simulink model "test"  (R2013b)
settings: Solver=ode45  StartTime=0.0  StopTime=10  RelTol=1e-3
settings Model: Creator=Walter  LastModifiedBy=Walter
settings DataIOCC: SignalLoggingSaveFormat=ModelDataLogs
settings DebuggingCC: MultiTaskDSMMsg=warning  MultiTaskCondExecSysMsg=none
settings RTWCC: IncludeERTFirstTime=on

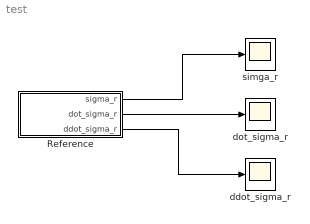
== system test ==
  Reference : Subsystem
  ddot_sigma_r : Scope
      settings: SaveName=ScopeData2
  dot_sigma_r : Scope
  simga_r : Scope
  wires:
  Reference/1(sigma_r) -> simga_r/1
  Reference/3(ddot_sigma_r) -> ddot_sigma_r/1
  Reference/2(dot_sigma_r) -> dot_sigma_r/1

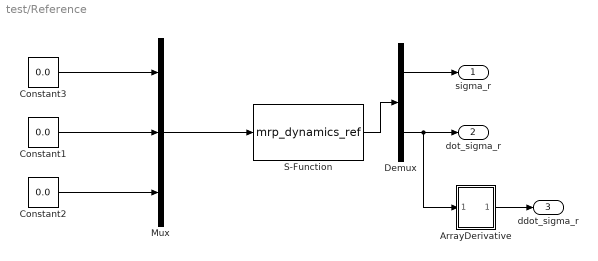
== system test/Reference ==
  ArrayDerivative : Subsystem
  Constant1 : Constant  Value=0.0
  Constant2 : Constant  Value=0.0
  Constant3 : Constant  Value=0.0
  Demux : Demux  Outputs=2
  Mux : Mux  Inputs=3
  S-Function : S-Function  FunctionName=mrp_dynamics_ref  EnableBusSupport=off
  sigma_r : Outport  PortDimensions=3
  dot_sigma_r : Outport  Port=2
  ddot_sigma_r : Outport  Port=3
  wires:
  Constant3/1 -> Mux/1
  Constant1/1 -> Mux/2
  Constant2/1 -> Mux/3
  Mux/1 -> S-Function/1
  S-Function/1 -> Demux/1
  Demux/1 -> sigma_r/1
  Demux/2 -> dot_sigma_r/1, ArrayDerivative/1(In1)
  ArrayDerivative/1(Out1) -> ddot_sigma_r/1

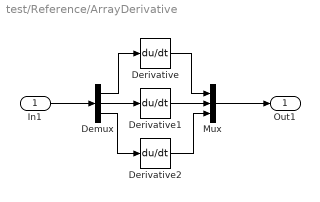
== system test/Reference/ArrayDerivative ==
  In1 : Inport
  Demux : Demux  Outputs=3
  Derivative : Derivative
  Derivative1 : Derivative
  Derivative2 : Derivative
  Mux : Mux  Inputs=3
  Out1 : Outport
  wires:
  Mux/1 -> Out1/1
  In1/1 -> Demux/1
  Derivative1/1 -> Mux/2
  Demux/2 -> Derivative1/1
  Derivative2/1 -> Mux/3
  Demux/3 -> Derivative2/1
  Demux/1 -> Derivative/1
  Derivative/1 -> Mux/1
